simulink library "AeroLoads"  (R2024a)
settings: Solver=VariableStepAuto  StartTime=0.0  StopTime=10.0  RelTol=1e-3
undefined symbols (not defined in the file): aero, geo
libraries: aerolibasang x3, simulink_extras x2, aerolibtransform2 x1, aerolibatmos2 x1
settings Model: Creator=igmso  LastModifiedBy=igmso

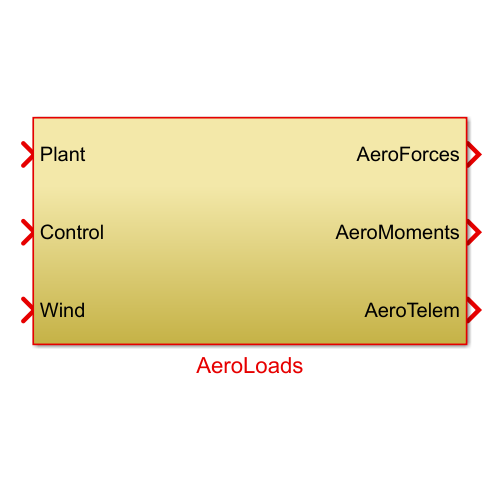
[thumbnail: Simulink's stored preview of the top-level diagram]
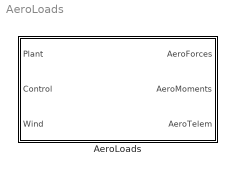
== system AeroLoads ==
  AeroLoads : Subsystem

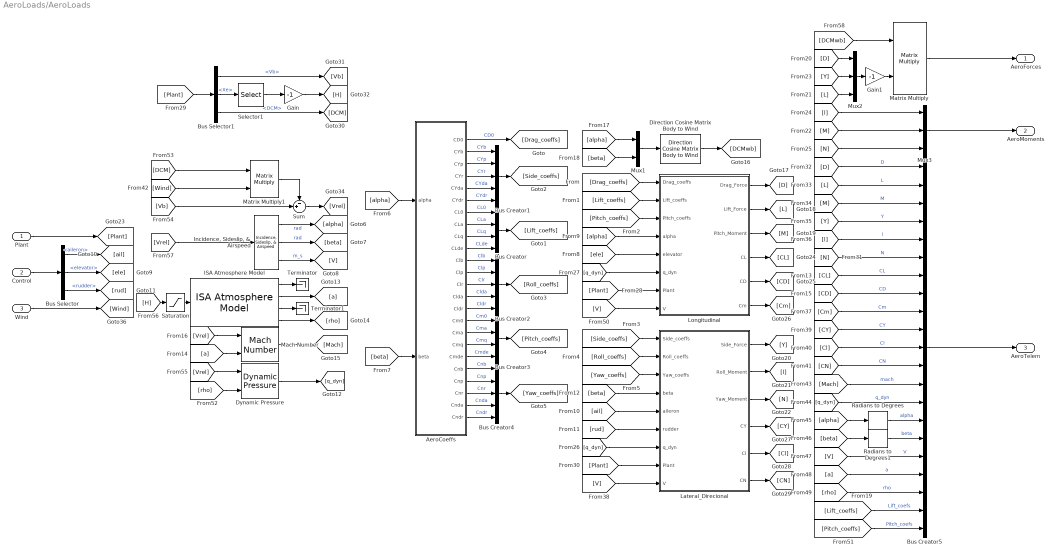
== system AeroLoads/AeroLoads ==
  Plant : Inport
  Control : Inport  Port=2
  Wind : Inport  Port=3
  AeroCoeffs : Subsystem
  Bus Creator : BusCreator  Inputs=4
  Bus Creator1 : BusCreator  Inputs=5
  Bus Creator2 : BusCreator  Inputs=5
  Bus Creator3 : BusCreator  Inputs=4
  Bus Creator4 : BusCreator  Inputs=5
  Bus Creator5 : BusCreator  Inputs=21
  Bus Selector : BusSelector  OutputSignals=aileron,elevator,rudder
  Bus Selector1 : BusSelector  OutputSignals=Vb,Xe,DCM
  Direction Cosine Matrix Body to Wind : aerolibtransform2/Direction Cosine Matrix Body to Wind
  Dynamic Pressure : aerolibasang/Dynamic Pressure
  Gain : Gain  Gain=-1
  Gain1 : Gain  Gain=-1
  ISA Atmosphere Model : aerolibatmos2/ISA Atmosphere Model  useExtended=off  action=Warning  custom=off  viscosityOut=off  g=9.80665  gamma=1.4  R=287.0531  L=0.0065  h_trop=11000  h_strat=20000  rho0=1.225  P0=101325  T0=288.15  h0=0  S=110.4  Tref=273.15  muref=1.716e-5
  "Incidence, Sideslip, & Airspeed" : aerolibasang/Incidence, Sideslip, & Airspeed
  Lateral_Direcional : Subsystem
  Longitudinal : Subsystem
  Mach Number : aerolibasang/Mach Number
  Matrix Multiply : Product  Multiplication=Matrix(*)
  Matrix Multiply1 : Product  Multiplication=Matrix(*)
  Mux1 : Mux  Inputs=2
  Mux2 : Mux  Inputs=3
  Mux3 : Mux  Inputs=3
  Radians to Degrees : simulink_extras/Transformations/Radians to Degrees
  Radians to Degrees1 : simulink_extras/Transformations/Radians to Degrees
  Saturation : Saturate  UpperLimit=20e3  LowerLimit=0
  Selector1 : Selector  InputPortWidth=3  IndexOptions=Index vector (dialog)  Indices=3  OutputSizes=1
  Sum : Sum  Inputs=-+|
  Terminator : Terminator
  Terminator1 : Terminator
  AeroForces : Outport
  AeroMoments : Outport  Port=2
  AeroTelem : Outport  Port=3
  wires:
  Matrix Multiply1/1 -> Sum/1
  [DCM] -> Matrix Multiply1/1
  Bus Selector1/3 -> [DCM]  "<DCM>"
  [Pitch_coeffs] -> Bus Creator5/21  "Pitch_coefs"
  [Lift_coeffs] -> Bus Creator5/20  "Lift_coefs"
  Mux3/1 -> AeroMoments/1
  Matrix Multiply/1 -> AeroForces/1
  Saturation/1 -> ISA Atmosphere Model/1
  Wind/1 -> [Wind]
  [rho] -> Dynamic Pressure/2
  Lateral_Direcional/6(CN) -> [CN]
  Lateral_Direcional/5(Cl) -> [Cl]
  Lateral_Direcional/4(CY) -> [CY]
  [Y] -> Mux2/2
  [V] -> Lateral_Direcional/9(V)
  Longitudinal/6(Cm) -> [Cm]
  Longitudinal/5(CD) -> [CD]
  Longitudinal/4(CL) -> [CL]
  [V] -> Longitudinal/8(V)
  Radians to Degrees1/1 -> Bus Creator5/16  "beta"
  Radians to Degrees/1 -> Bus Creator5/15  "alpha"
  Control/1 -> Bus Selector/1
  Plant/1 -> [Plant]
  [CL] -> Bus Creator5/7  "CL"
  [N] -> Bus Creator5/6  "N"
  [CD] -> Bus Creator5/8  "CD"
  [Y] -> Bus Creator5/4  "Y"
  [D] -> Bus Creator5/1  "D"
  [M] -> Bus Creator5/3  "M"
  [L] -> Bus Creator5/2  "L"
  Direction Cosine Matrix Body to Wind/1 -> [DCMwb]
  [beta] -> Mux1/2
  [D] -> Mux2/1
  Lateral_Direcional/3(Yaw_Moment) -> [N]
  Lateral_Direcional/2(Roll_Moment) -> [l]
  Lateral_Direcional/1(Side_Force) -> [Y]
  Gain1/1 -> Matrix Multiply/2
  Longitudinal/1(Drag_Force) -> [D]
  [L] -> Mux2/3
  [q_dyn] -> Lateral_Direcional/7(q_dyn)
  Longitudinal/3(Pitch_Moment) -> [M]
  [q_dyn] -> Longitudinal/6(q_dyn)
  "Incidence, Sideslip, & Airspeed"/1 -> [alpha]  "rad"
  "Incidence, Sideslip, & Airspeed"/2 -> [beta]  "rad"
  ISA Atmosphere Model/3 -> Terminator1/1
  ISA Atmosphere Model/2 -> [a]
  Bus Creator5/1 -> AeroTelem/1
  [a] -> Bus Creator5/18  "a"
  [V] -> Bus Creator5/17  "V"
  Mux1/1 -> Direction Cosine Matrix Body to Wind/1
  [alpha] -> Radians to Degrees/1
  [CN] -> Bus Creator5/12  "CN"
  [CY] -> Bus Creator5/10  "CY"
  [alpha] -> Mux1/1
  [q_dyn] -> Bus Creator5/14  "q_dyn"
  Bus Selector/3 -> [rud]  "<rudder>"
  Mux2/1 -> Gain1/1
  "Incidence, Sideslip, & Airspeed"/3 -> [V]  "m_s"
  [ail] -> Lateral_Direcional/5(aileron)
  AeroCoeffs/1(CD0) -> [Drag_coeffs]  "CD0"
  [alpha] -> Longitudinal/4(alpha)
  [rud] -> Lateral_Direcional/6(rudder)
  [N] -> Mux3/3
  [beta] -> Lateral_Direcional/4(beta)
  [Pitch_coeffs] -> Longitudinal/3(Pitch_coeffs)
  [a] -> Mach Number/2
  [Lift_coeffs] -> Longitudinal/2(Lift_coeffs)
  AeroCoeffs/23(Cnda) -> Bus Creator4/4  "Cnda"
  [Roll_coeffs] -> Lateral_Direcional/2(Roll_coeffs)
  AeroCoeffs/24(Cndr) -> Bus Creator4/5  "Cndr"
  [Drag_coeffs] -> Longitudinal/1(Drag_coeffs)
  Bus Selector/2 -> [ele]  "<elevator>"
  [Cm] -> Bus Creator5/9  "Cm"
  Bus Creator/1 -> [Lift_coeffs]
  [alpha] -> AeroCoeffs/1(alpha)
  AeroCoeffs/8(CLa) -> Bus Creator/2  "CLa"
  [M] -> Mux3/2
  AeroCoeffs/4(CYr) -> Bus Creator1/3  "CYr"
  AeroCoeffs/2(CYb) -> Bus Creator1/1  "CYb"
  Dynamic Pressure/1 -> [q_dyn]
  [DCMwb] -> Matrix Multiply/1
  [Plant] -> Lateral_Direcional/8(Plant)
  [l] -> Mux3/1
  ISA Atmosphere Model/4 -> [rho]
  AeroCoeffs/11(Clb) -> Bus Creator2/1  "Clb"
  AeroCoeffs/12(Clp) -> Bus Creator2/2  "Clp"
  [l] -> Bus Creator5/5  "l"
  AeroCoeffs/13(Clr) -> Bus Creator2/3  "Clr"
  [Side_coeffs] -> Lateral_Direcional/1(Side_coeffs)
  AeroCoeffs/15(Cldr) -> Bus Creator2/5  "Cldr"
  ISA Atmosphere Model/1 -> Terminator/1
  AeroCoeffs/9(CLq) -> Bus Creator/3  "CLq"
  Bus Creator2/1 -> [Roll_coeffs]
  [ele] -> Longitudinal/5(elevator)
  AeroCoeffs/14(Clda) -> Bus Creator2/4  "Clda"
  AeroCoeffs/3(CYp) -> Bus Creator1/2  "CYp"
  AeroCoeffs/21(Cnp) -> Bus Creator4/2  "Cnp"
  AeroCoeffs/22(Cnr) -> Bus Creator4/3  "Cnr"
  [Mach] -> Bus Creator5/13  "mach"
  Mach Number/1 -> [Mach]
  Bus Creator4/1 -> [Yaw_coeffs]
  AeroCoeffs/5(CYda) -> Bus Creator1/4  "CYda"
  [H] -> Saturation/1
  AeroCoeffs/17(Cma) -> Bus Creator3/2  "Cma"
  AeroCoeffs/18(Cmq) -> Bus Creator3/3  "Cmq"
  [Cl] -> Bus Creator5/11  "Cl"
  [rho] -> Bus Creator5/19  "rho"
  AeroCoeffs/7(CL0) -> Bus Creator/1  "CL0"
  AeroCoeffs/16(Cm0) -> Bus Creator3/1  "Cm0"
  AeroCoeffs/19(Cmde) -> Bus Creator3/4  "Cmde"
  [Yaw_coeffs] -> Lateral_Direcional/3(Yaw_coeffs)
  Bus Creator1/1 -> [Side_coeffs]
  [Plant] -> Longitudinal/7(Plant)
  AeroCoeffs/6(CYdr) -> Bus Creator1/5  "CYdr"
  AeroCoeffs/10(CLde) -> Bus Creator/4  "CLde"
  AeroCoeffs/20(Cnb) -> Bus Creator4/1  "Cnb"
  [beta] -> AeroCoeffs/2(beta)
  [beta] -> Radians to Degrees1/1
  Bus Creator3/1 -> [Pitch_coeffs]
  Longitudinal/2(Lift_Force) -> [L]
  Bus Selector/1 -> [ail]  "<aileron>"
  [Vrel] -> "Incidence, Sideslip, & Airspeed"/1
  [Vrel] -> Mach Number/1
  [Vrel] -> Dynamic Pressure/1
  Bus Selector1/2 -> Selector1/1  "<Xe>"
  Selector1/1 -> Gain/1
  Gain/1 -> [H]
  [Plant] -> Bus Selector1/1
  Bus Selector1/1 -> [Vb]  "<Vb>"
  [Vb] -> Sum/2
  Sum/1 -> [Vrel]
  [Wind] -> Matrix Multiply1/2

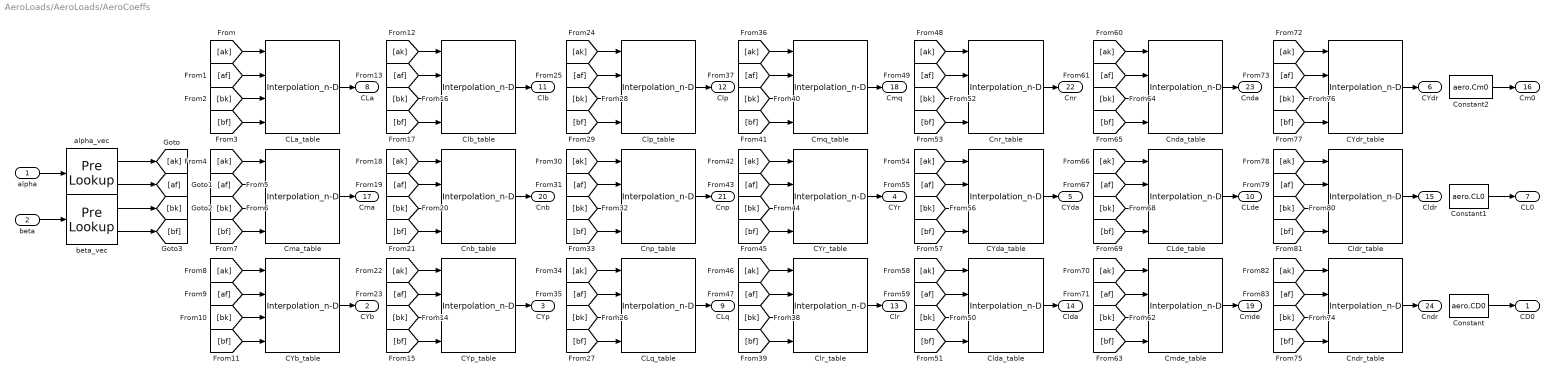
== system AeroLoads/AeroLoads/AeroCoeffs ==
  alpha : Inport
  beta : Inport  Port=2
  CLa_table : Interpolation_n-D  Table=reshape(aero.CLa,23,[])  ExtrapMethod=Clip  InternalRulePriority=Speed
  CLde_table : Interpolation_n-D  Table=reshape(aero.CLd02,23,[])  ExtrapMethod=Clip  InternalRulePriority=Speed
  CLq_table : Interpolation_n-D  Table=reshape(aero.CLq,23,[])  ExtrapMethod=Clip  InternalRulePriority=Speed
  CYb_table : Interpolation_n-D  Table=reshape(aero.CYb,23,[])  ExtrapMethod=Clip  InternalRulePriority=Speed
  CYda_table : Interpolation_n-D  Table=reshape(aero.CYd01,23,[])  ExtrapMethod=Clip  InternalRulePriority=Speed
  CYdr_table : Interpolation_n-D  Table=reshape(aero.CYd03,23,[])  ExtrapMethod=Clip  InternalRulePriority=Speed
  CYp_table : Interpolation_n-D  Table=reshape(aero.CYp,23,[])  ExtrapMethod=Clip  InternalRulePriority=Speed
  CYr_table : Interpolation_n-D  Table=reshape(aero.CYr,23,[])  ExtrapMethod=Clip  InternalRulePriority=Speed
  Clb_table : Interpolation_n-D  Table=reshape(aero.Clb,23,[])  ExtrapMethod=Clip  InternalRulePriority=Speed
  Clda_table : Interpolation_n-D  Table=reshape(aero.Cld01,23,[])  ExtrapMethod=Clip  InternalRulePriority=Speed
  Cldr_table : Interpolation_n-D  Table=reshape(aero.Cld03,23,[])  ExtrapMethod=Clip  InternalRulePriority=Speed
  Clp_table : Interpolation_n-D  Table=reshape(aero.Clp,23,[])  ExtrapMethod=Clip  InternalRulePriority=Speed
  Clr_table : Interpolation_n-D  Table=reshape(aero.Clr,23,[])  ExtrapMethod=Clip  InternalRulePriority=Speed
  Cma_table : Interpolation_n-D  Table=reshape(aero.Cma,23,[])  ExtrapMethod=Clip  InternalRulePriority=Speed
  Cmde_table : Interpolation_n-D  Table=reshape(aero.Cmd02,23,[])  ExtrapMethod=Clip  InternalRulePriority=Speed
  Cmq_table : Interpolation_n-D  Table=reshape(aero.Cmq,23,[])  ExtrapMethod=Clip  InternalRulePriority=Speed
  Cnb_table : Interpolation_n-D  Table=reshape(aero.Cnb,23,[])  ExtrapMethod=Clip  InternalRulePriority=Speed
  Cnda_table : Interpolation_n-D  Table=reshape(aero.Cnd01,23,[])  ExtrapMethod=Clip  InternalRulePriority=Speed
  Cndr_table : Interpolation_n-D  Table=reshape(aero.Cnd03,23,[])  ExtrapMethod=Clip  InternalRulePriority=Speed
  Cnp_table : Interpolation_n-D  Table=reshape(aero.Cnp,23,[])  ExtrapMethod=Clip  InternalRulePriority=Speed
  Cnr_table : Interpolation_n-D  Table=reshape(aero.Cnr,23,[])  ExtrapMethod=Clip  InternalRulePriority=Speed
  Constant : Constant  Value=aero.CD0  SampleTime=-1
  Constant1 : Constant  Value=aero.CL0  SampleTime=-1
  Constant2 : Constant  Value=aero.Cm0  SampleTime=-1
  alpha_vec : PreLookup  BreakpointsData=-10:1:12
  beta_vec : PreLookup  BreakpointsData=-5:1:5
  CD0 : Outport
  CYb : Outport  Port=2
  CYp : Outport  Port=3
  CYr : Outport  Port=4
  CYda : Outport  Port=5
  CYdr : Outport  Port=6
  CL0 : Outport  Port=7
  CLa : Outport  Port=8
  CLq : Outport  Port=9
  CLde : Outport  Port=10
  Clb : Outport  Port=11
  Clp : Outport  Port=12
  Clr : Outport  Port=13
  Clda : Outport  Port=14
  Cldr : Outport  Port=15
  Cm0 : Outport  Port=16
  Cma : Outport  Port=17
  Cmq : Outport  Port=18
  Cmde : Outport  Port=19
  Cnb : Outport  Port=20
  Cnp : Outport  Port=21
  Cnr : Outport  Port=22
  Cnda : Outport  Port=23
  Cndr : Outport  Port=24
  wires:
  Constant/1 -> CD0/1
  Constant1/1 -> CL0/1
  Constant2/1 -> Cm0/1
  alpha_vec/1 -> [ak]
  alpha_vec/2 -> [af]
  alpha/1 -> alpha_vec/1
  beta_vec/1 -> [bk]
  beta/1 -> beta_vec/1
  beta_vec/2 -> [bf]
  CLq_table/1 -> CLq/1
  CYdr_table/1 -> CYdr/1
  Cndr_table/1 -> Cndr/1
  CLde_table/1 -> CLde/1
  Cmde_table/1 -> Cmde/1
  CYb_table/1 -> CYb/1
  Clda_table/1 -> Clda/1
  CYda_table/1 -> CYda/1
  Cmq_table/1 -> Cmq/1
  Cnr_table/1 -> Cnr/1
  Cnb_table/1 -> Cnb/1
  CLa_table/1 -> CLa/1
  [bk] -> Cndr_table/3
  [ak] -> Cldr_table/1
  [ak] -> Cndr_table/1
  Cma_table/1 -> Cma/1
  [bf] -> Cndr_table/4
  [af] -> Cldr_table/2
  [ak] -> CYdr_table/1
  [bk] -> CYdr_table/3
  Cldr_table/1 -> Cldr/1
  [af] -> CYdr_table/2
  [ak] -> CLq_table/1
  [af] -> CLq_table/2
  Clr_table/1 -> Clr/1
  [bf] -> CLq_table/4
  [af] -> Cnp_table/2
  [bk] -> Cnp_table/3
  [bf] -> Clp_table/4
  [bk] -> Clp_table/3
  [bf] -> Cnp_table/4
  [bk] -> CLq_table/3
  [bk] -> CLde_table/3
  [ak] -> Cmde_table/1
  [af] -> Cmde_table/2
  [ak] -> Clb_table/1
  Clp_table/1 -> Clp/1
  [af] -> Cnda_table/2
  [bk] -> Clr_table/3
  CYp_table/1 -> CYp/1
  [af] -> Cndr_table/2
  [bk] -> Cmq_table/3
  Cnp_table/1 -> Cnp/1
  [ak] -> Clp_table/1
  [ak] -> Cnp_table/1
  [bf] -> Cnb_table/4
  [bf] -> CYr_table/4
  [bk] -> Clb_table/3
  [af] -> Cnb_table/2
  [bk] -> Cmde_table/3
  [af] -> Clr_table/2
  Clb_table/1 -> Clb/1
  [bf] -> CYdr_table/4
  [bk] -> Cnda_table/3
  CYr_table/1 -> CYr/1
  [bf] -> Clda_table/4
  [ak] -> Clr_table/1
  [bf] -> Cldr_table/4
  [ak] -> Cmq_table/1
  [bf] -> Cmde_table/4
  [af] -> Clda_table/2
  [bk] -> CYb_table/3
  [af] -> CYda_table/2
  [bf] -> Cmq_table/4
  [bf] -> CYb_table/4
  [bf] -> Clr_table/4
  [bf] -> CLde_table/4
  [ak] -> CLde_table/1
  [bf] -> CYp_table/4
  [af] -> CYp_table/2
  [af] -> Cnr_table/2
  [bf] -> CYda_table/4
  [bf] -> Cnr_table/4
  [bf] -> Clb_table/4
  [bk] -> Cnr_table/3
  [ak] -> Cnr_table/1
  [ak] -> Clda_table/1
  [af] -> Clp_table/2
  [ak] -> CYda_table/1
  [ak] -> CYr_table/1
  [af] -> CYb_table/2
  [ak] -> Cnda_table/1
  [af] -> Cmq_table/2
  [bk] -> CYr_table/3
  [ak] -> CLa_table/1
  [bf] -> CLa_table/4
  [af] -> CLa_table/2
  [ak] -> CYp_table/1
  [bk] -> Cma_table/3
  Cnda_table/1 -> Cnda/1
  [af] -> CLde_table/2
  [bk] -> Cldr_table/3
  [ak] -> Cma_table/1
  [bk] -> Cnb_table/3
  [af] -> Clb_table/2
  [bf] -> Cma_table/4
  [af] -> CYr_table/2
  [bf] -> Cnda_table/4
  [ak] -> CYb_table/1
  [af] -> Cma_table/2
  [ak] -> Cnb_table/1
  [bk] -> CLa_table/3
  [bk] -> Clda_table/3
  [bk] -> CYda_table/3
  [bk] -> CYp_table/3

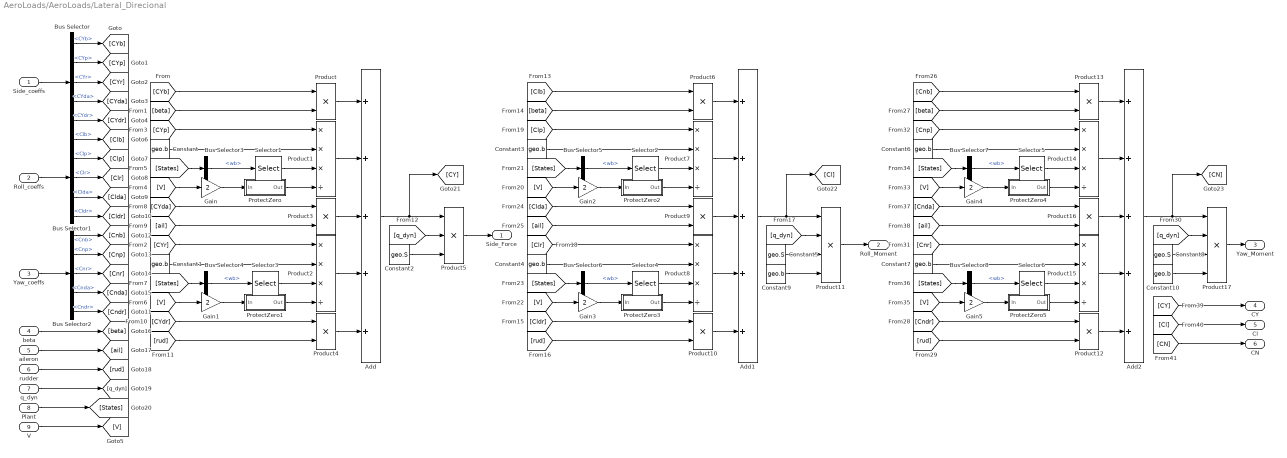
== system AeroLoads/AeroLoads/Lateral_Direcional ==
  Side_coeffs : Inport
  Roll_coeffs : Inport  Port=2
  Yaw_coeffs : Inport  Port=3
  beta : Inport  Port=4
  aileron : Inport  Port=5
  rudder : Inport  Port=6
  q_dyn : Inport  Port=7
  Plant : Inport  Port=8
  V : Inport  Port=9
  Add : Sum  Inputs=5
  Add1 : Sum  Inputs=5
  Add2 : Sum  Inputs=5
  Bus Selector : BusSelector  OutputSignals=CYb,CYp,CYr,CYda,CYdr
  Bus Selector1 : BusSelector  OutputSignals=Clb,Clp,Clr,Clda,Cldr
  Bus Selector2 : BusSelector  OutputSignals=Cnb,Cnp,Cnr,Cnda,Cndr
  Bus Selector{3..8} (6 alike) : BusSelector  OutputSignals=wb
  Constant{,1,3..4,6..7,9..10} (8 alike) : Constant  Value=geo.b  SampleTime=-1
  Constant2 : Constant  Value=geo.S  SampleTime=-1
  Constant5 : Constant  Value=geo.S  SampleTime=-1
  Constant8 : Constant  Value=geo.S  SampleTime=-1
  Gain{,1..5} (6 alike) : Gain  Gain=2
  Product{,3..4,6,9..10,12..13,16} (9 alike) : Product
  Product{1..2,7..8,14..15} (6 alike) : Product  Inputs=***/
  Product11 : Product  Inputs=4
  Product17 : Product  Inputs=4
  Product5 : Product  Inputs=3
  ProtectZero : Subsystem
  ProtectZero1 : Subsystem
  ProtectZero2 : Subsystem
  ProtectZero3 : Subsystem
  ProtectZero4 : Subsystem
  ProtectZero5 : Subsystem
  Selector1 : Selector  InputPortWidth=3  IndexOptions=Index vector (dialog)  Indices=1  OutputSizes=1
  Selector2 : Selector  InputPortWidth=3  IndexOptions=Index vector (dialog)  Indices=1  OutputSizes=1
  Selector3 : Selector  InputPortWidth=3  IndexOptions=Index vector (dialog)  Indices=3  OutputSizes=1
  Selector4 : Selector  InputPortWidth=3  IndexOptions=Index vector (dialog)  Indices=3  OutputSizes=1
  Selector5 : Selector  InputPortWidth=3  IndexOptions=Index vector (dialog)  Indices=1  OutputSizes=1
  Selector6 : Selector  InputPortWidth=3  IndexOptions=Index vector (dialog)  Indices=3  OutputSizes=1
  Side_Force : Outport
  Roll_Moment : Outport  Port=2
  Yaw_Moment : Outport  Port=3
  CY : Outport  Port=4
  Cl : Outport  Port=5
  CN : Outport  Port=6
  wires:
  [CN] -> CN/1
  [Cl] -> Cl/1
  [CY] -> CY/1
  Product17/1 -> Yaw_Moment/1
  Constant10/1 -> Product17/4
  Constant9/1 -> Product11/4
  [q_dyn] -> Product17/2
  Constant8/1 -> Product17/3
  Add2/1 -> [CN], Product17/1
  Product15/1 -> Add2/4
  ProtectZero5/1(Out) -> Product15/4
  [Cnr] -> Product15/1
  Bus Selector8/1 -> Selector6/1  "<wb>"
  Constant7/1 -> Product15/2
  [States] -> Bus Selector8/1
  Gain5/1 -> ProtectZero5/1(In)
  [V] -> Gain5/1
  Product13/1 -> Add2/1
  Product14/1 -> Add2/2
  Product12/1 -> Add2/5
  Product16/1 -> Add2/3
  [rud] -> Product12/2
  [Cndr] -> Product12/1
  [Cnda] -> Product16/1
  [ail] -> Product16/2
  [beta] -> Product13/2
  [Cnb] -> Product13/1
  Constant6/1 -> Product14/2
  ProtectZero4/1(Out) -> Product14/4
  [Cnp] -> Product14/1
  Bus Selector7/1 -> Selector5/1  "<wb>"
  [V] -> Gain4/1
  [States] -> Bus Selector7/1
  Gain4/1 -> ProtectZero4/1(In)
  Gain2/1 -> ProtectZero2/1(In)
  [States] -> Bus Selector5/1
  [V] -> Gain2/1
  Bus Selector5/1 -> Selector2/1  "<wb>"
  [Clp] -> Product7/1
  ProtectZero2/1(Out) -> Product7/4
  Constant3/1 -> Product7/2
  [Clb] -> Product6/1
  [beta] -> Product6/2
  [ail] -> Product9/2
  [Clda] -> Product9/1
  [Cldr] -> Product10/1
  [rud] -> Product10/2
  Product9/1 -> Add1/3
  Product10/1 -> Add1/5
  Product7/1 -> Add1/2
  Product6/1 -> Add1/1
  [V] -> Gain3/1
  Gain3/1 -> ProtectZero3/1(In)
  [States] -> Bus Selector6/1
  Constant4/1 -> Product8/2
  Bus Selector6/1 -> Selector4/1  "<wb>"
  [Clr] -> Product8/1
  ProtectZero3/1(Out) -> Product8/4
  Product8/1 -> Add1/4
  Add1/1 -> [Cl], Product11/1
  Constant5/1 -> Product11/3
  [q_dyn] -> Product11/2
  Product11/1 -> Roll_Moment/1
  Product5/1 -> Side_Force/1
  [q_dyn] -> Product5/2
  Constant2/1 -> Product5/3
  Add/1 -> Product5/1, [CY]
  Product2/1 -> Add/4
  ProtectZero1/1(Out) -> Product2/4
  [CYr] -> Product2/1
  Bus Selector4/1 -> Selector3/1  "<wb>"
  Constant1/1 -> Product2/2
  [States] -> Bus Selector4/1
  Gain1/1 -> ProtectZero1/1(In)
  [V] -> Gain1/1
  Product/1 -> Add/1
  Product1/1 -> Add/2
  Product4/1 -> Add/5
  Product3/1 -> Add/3
  [rud] -> Product4/2
  [CYdr] -> Product4/1
  [CYda] -> Product3/1
  [ail] -> Product3/2
  [beta] -> Product/2
  [CYb] -> Product/1
  Constant/1 -> Product1/2
  ProtectZero/1(Out) -> Product1/4
  [CYp] -> Product1/1
  Bus Selector3/1 -> Selector1/1  "<wb>"
  [V] -> Gain/1
  [States] -> Bus Selector3/1
  Gain/1 -> ProtectZero/1(In)
  Plant/1 -> [States]
  q_dyn/1 -> [q_dyn]
  rudder/1 -> [rud]
  aileron/1 -> [ail]
  beta/1 -> [beta]
  Yaw_coeffs/1 -> Bus Selector2/1
  Bus Selector2/3 -> [Cnr]  "<Cnr>"
  Bus Selector2/2 -> [Cnp]  "<Cnp>"
  Bus Selector2/4 -> [Cnda]  "<Cnda>"
  Bus Selector2/1 -> [Cnb]  "<Cnb>"
  Bus Selector2/5 -> [Cndr]  "<Cndr>"
  Bus Selector1/5 -> [Cldr]  "<Cldr>"
  Bus Selector1/1 -> [Clb]  "<Clb>"
  Bus Selector1/4 -> [Clda]  "<Clda>"
  Bus Selector1/2 -> [Clp]  "<Clp>"
  Bus Selector1/3 -> [Clr]  "<Clr>"
  Roll_coeffs/1 -> Bus Selector1/1
  Bus Selector/5 -> [CYdr]  "<CYdr>"
  Bus Selector/4 -> [CYda]  "<CYda>"
  Bus Selector/3 -> [CYr]  "<CYr>"
  Bus Selector/2 -> [CYp]  "<CYp>"
  Bus Selector/1 -> [CYb]  "<CYb>"
  Side_coeffs/1 -> Bus Selector/1
  V/1 -> [V]
  Selector1/1 -> Product1/3
  Selector2/1 -> Product7/3
  Selector3/1 -> Product2/3
  Selector4/1 -> Product8/3
  Selector6/1 -> Product15/3
  Selector5/1 -> Product14/3

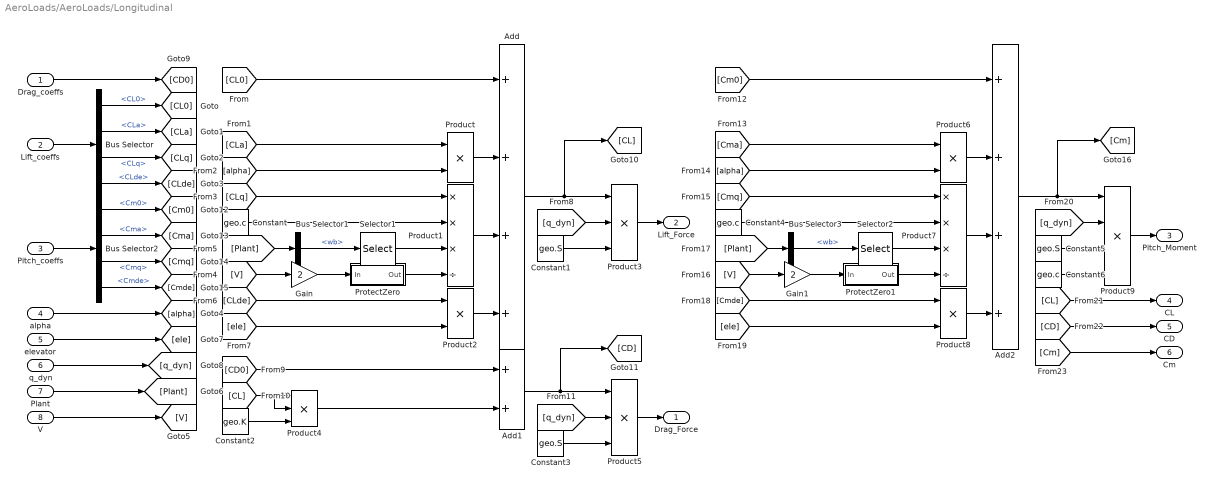
== system AeroLoads/AeroLoads/Longitudinal ==
  Drag_coeffs : Inport
  Lift_coeffs : Inport  Port=2
  Pitch_coeffs : Inport  Port=3
  alpha : Inport  Port=4
  elevator : Inport  Port=5
  q_dyn : Inport  Port=6
  Plant : Inport  Port=7
  V : Inport  Port=8
  Add : Sum  Inputs=4
  Add1 : Sum
  Add2 : Sum  Inputs=4
  Bus Selector : BusSelector  OutputSignals=CL0,CLa,CLq,CLde
  Bus Selector1 : BusSelector  OutputSignals=wb
  Bus Selector2 : BusSelector  OutputSignals=Cm0,Cma,Cmq,Cmde
  Bus Selector3 : BusSelector  OutputSignals=wb
  Constant : Constant  Value=geo.c  SampleTime=-1
  Constant1 : Constant  Value=geo.S  SampleTime=-1
  Constant2 : Constant  Value=geo.K  SampleTime=-1
  Constant3 : Constant  Value=geo.S  SampleTime=-1
  Constant4 : Constant  Value=geo.c  SampleTime=-1
  Constant5 : Constant  Value=geo.S  SampleTime=-1
  Constant6 : Constant  Value=geo.c  SampleTime=-1
  Gain : Gain  Gain=2
  Gain1 : Gain  Gain=2
  Product{,2,6,8} (4 alike) : Product
  Product1 : Product  Inputs=***/
  Product3 : Product  Inputs=3
  Product4 : Product  Inputs=3
  Product5 : Product  Inputs=3
  Product7 : Product  Inputs=***/
  Product9 : Product  Inputs=4
  ProtectZero : Subsystem
  ProtectZero1 : Subsystem
  Selector1 : Selector  InputPortWidth=3  IndexOptions=Index vector (dialog)  Indices=2  OutputSizes=1
  Selector2 : Selector  InputPortWidth=3  IndexOptions=Index vector (dialog)  Indices=2  OutputSizes=1
  Drag_Force : Outport
  Lift_Force : Outport  Port=2
  Pitch_Moment : Outport  Port=3
  CL : Outport  Port=4
  CD : Outport  Port=5
  Cm : Outport  Port=6
  wires:
  Constant6/1 -> Product9/4
  [Cm] -> Cm/1
  [CD] -> CD/1
  [CL] -> CL/1
  [ele] -> Product8/2
  [Cma] -> Product6/1
  [alpha] -> Product6/2
  [Plant] -> Bus Selector3/1
  Bus Selector3/1 -> Selector2/1  "<wb>"
  [Cmq] -> Product7/1
  Constant4/1 -> Product7/2
  [V] -> Gain1/1
  Gain1/1 -> ProtectZero1/1(In)
  ProtectZero1/1(Out) -> Product7/4
  [Cmde] -> Product8/1
  [Cm0] -> Add2/1
  Product6/1 -> Add2/2
  Product7/1 -> Add2/3
  Product8/1 -> Add2/4
  Add2/1 -> [Cm], Product9/1
  [q_dyn] -> Product9/2
  Constant5/1 -> Product9/3
  Product9/1 -> Pitch_Moment/1
  Bus Selector2/1 -> [Cm0]  "<Cm0>"
  Bus Selector2/2 -> [Cma]  "<Cma>"
  Bus Selector2/3 -> [Cmq]  "<Cmq>"
  Bus Selector2/4 -> [Cmde]  "<Cmde>"
  Pitch_coeffs/1 -> Bus Selector2/1
  [q_dyn] -> Product5/2
  Product5/1 -> Drag_Force/1
  Add1/1 -> Product5/1, [CD]
  Constant3/1 -> Product5/3
  Product4/1 -> Add1/2
  [CD0] -> Add1/1
  Constant2/1 -> Product4/3
  [CL] -> Product4/1, Product4/2
  Drag_coeffs/1 -> [CD0]
  Product3/1 -> Lift_Force/1
  Constant1/1 -> Product3/3
  [q_dyn] -> Product3/2
  q_dyn/1 -> [q_dyn]
  Add/1 -> Product3/1, [CL]
  Product2/1 -> Add/4
  Product1/1 -> Add/3
  Product/1 -> Add/2
  [CL0] -> Add/1
  [ele] -> Product2/2
  elevator/1 -> [ele]
  [CLde] -> Product2/1
  ProtectZero/1(Out) -> Product1/4
  Gain/1 -> ProtectZero/1(In)
  [V] -> Gain/1
  Constant/1 -> Product1/2
  [CLq] -> Product1/1
  Bus Selector1/1 -> Selector1/1  "<wb>"
  [Plant] -> Bus Selector1/1
  Plant/1 -> [Plant]
  V/1 -> [V]
  [alpha] -> Product/2
  alpha/1 -> [alpha]
  [CLa] -> Product/1
  Bus Selector/4 -> [CLde]  "<CLde>"
  Bus Selector/3 -> [CLq]  "<CLq>"
  Bus Selector/2 -> [CLa]  "<CLa>"
  Bus Selector/1 -> [CL0]  "<CL0>"
  Lift_coeffs/1 -> Bus Selector/1
  Selector1/1 -> Product1/3
  Selector2/1 -> Product7/3

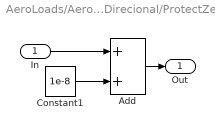
== system AeroLoads/AeroLoads/Lateral_Direcional/ProtectZero ==
  In : Inport
  Add : Sum
  Constant1 : Constant  Value=1e-8  SampleTime=-1
  Out : Outport
  wires:
  In/1 -> Add/1
  Add/1 -> Out/1
  Constant1/1 -> Add/2

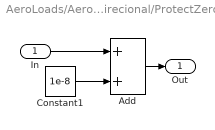
== system AeroLoads/AeroLoads/Lateral_Direcional/ProtectZero1 ==
  In : Inport
  Add : Sum
  Constant1 : Constant  Value=1e-8  SampleTime=-1
  Out : Outport
  wires:
  Constant1/1 -> Add/2
  Add/1 -> Out/1
  In/1 -> Add/1

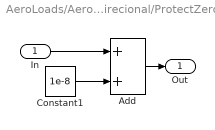
== system AeroLoads/AeroLoads/Lateral_Direcional/ProtectZero2 ==
  In : Inport
  Add : Sum
  Constant1 : Constant  Value=1e-8  SampleTime=-1
  Out : Outport
  wires:
  Constant1/1 -> Add/2
  Add/1 -> Out/1
  In/1 -> Add/1

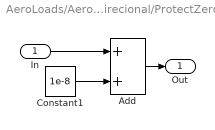
== system AeroLoads/AeroLoads/Lateral_Direcional/ProtectZero3 ==
  In : Inport
  Add : Sum
  Constant1 : Constant  Value=1e-8  SampleTime=-1
  Out : Outport
  wires:
  In/1 -> Add/1
  Add/1 -> Out/1
  Constant1/1 -> Add/2

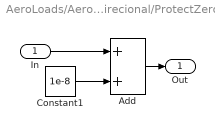
== system AeroLoads/AeroLoads/Lateral_Direcional/ProtectZero4 ==
  In : Inport
  Add : Sum
  Constant1 : Constant  Value=1e-8  SampleTime=-1
  Out : Outport
  wires:
  In/1 -> Add/1
  Add/1 -> Out/1
  Constant1/1 -> Add/2

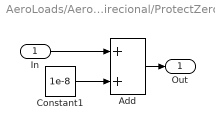
== system AeroLoads/AeroLoads/Lateral_Direcional/ProtectZero5 ==
  In : Inport
  Add : Sum
  Constant1 : Constant  Value=1e-8  SampleTime=-1
  Out : Outport
  wires:
  Constant1/1 -> Add/2
  Add/1 -> Out/1
  In/1 -> Add/1

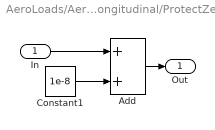
== system AeroLoads/AeroLoads/Longitudinal/ProtectZero ==
  In : Inport
  Add : Sum
  Constant1 : Constant  Value=1e-8  SampleTime=-1
  Out : Outport
  wires:
  In/1 -> Add/1
  Add/1 -> Out/1
  Constant1/1 -> Add/2

== system AeroLoads/AeroLoads/Longitudinal/ProtectZero1 ==
  In : Inport
  Add : Sum
  Constant1 : Constant  Value=1e-8  SampleTime=-1
  Out : Outport
  wires:
  Constant1/1 -> Add/2
  Add/1 -> Out/1
  In/1 -> Add/1
